simulink model "HILClimbers_LED_Rear_Light_Module_V5"  (R2021a)
settings: Solver=VariableStepAuto  StartTime=0.0  StopTime=inf  RelTol=1e-3
model workspace (MAT data in the model file):
  brake = 0
settings Model: Creator=Sai229  LastModifiedBy=Sai229

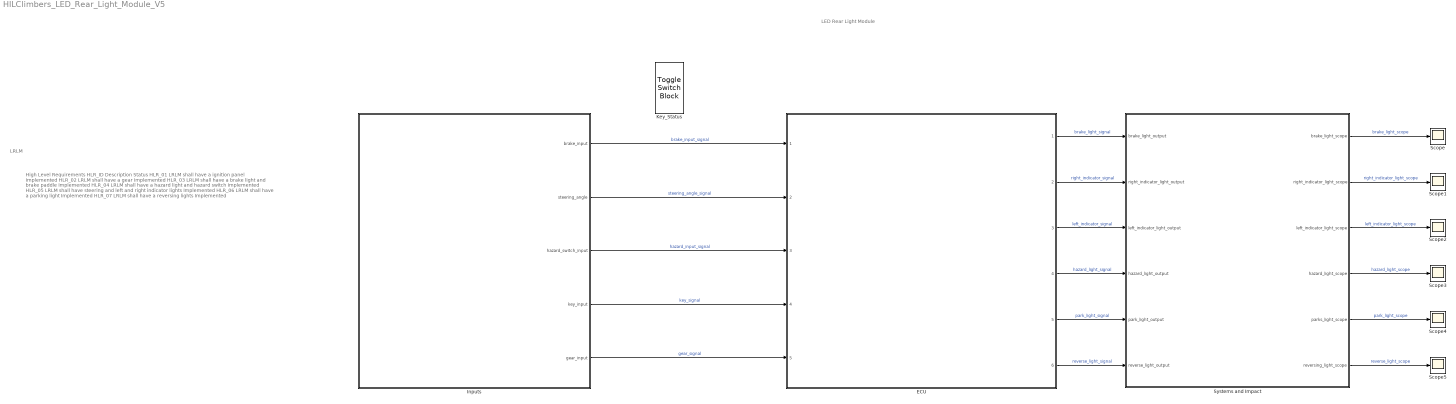
== system HILClimbers_LED_Rear_Light_Module_V5 ==
  note: LRLM
  note: High Level Requirements
      |
      | HLR_ID
      | Description
      | Status
      |
      | HLR_01
      | LRLM shall have a ignition panel
      | Implemented
      |
      | HLR_02
      | LRLM shall have a gear
      | Implemented
      |
      | HLR_03
      | LRLM shall have a brake light and brake paddle
      | Implemented
      |
      | HLR_04
      | LRLM shall have a hazard light and hazard switch
      | Implemented
      |
      | HLR_05
      | LRLM shall have steering and left and right indicator lights
      | Implemented
      |
      | HLR_06
      | LRLM shall have a parking light
      | Implemented
      |
      | HLR_07
      | LRLM shall have a reversing lights
      | Implemented
  note: LED Rear Light Module
  ECU : Subsystem  ReferencedSubsystem=LRLM_ECU
  Inputs : Subsystem
  Key_Status : ToggleSwitchBlock  LabelPosition=Hide
      settings: Values={{'Off', 'On'}, [0 1]}
  Scope{,1..5} (6 alike) : Scope
  Systems and Impact : Subsystem
  wires:
  Inputs/1(brake_input) -> ECU/1  "brake_input_signal"
  Inputs/2(steering_angle) -> ECU/2  "steering_angle_signal"
  Inputs/3(hazard_switch_input) -> ECU/3  "hazard_input_signal"
  Inputs/4(key_input) -> ECU/4  "key_signal"
  Inputs/5(gear_input) -> ECU/5  "gear_signal"
  ECU/1 -> Systems and Impact/1(brake_light_output)  "brake_light_signal"
  ECU/2 -> Systems and Impact/2(right_indicator_light_output)  "right_indicator_signal"
  ECU/3 -> Systems and Impact/3(left_indicator_light_output)  "left_indicator_signal"
  ECU/4 -> Systems and Impact/4(hazard_light_output)  "hazard_light_signal"
  ECU/5 -> Systems and Impact/5(park_light_output)  "park_light_signal"
  ECU/6 -> Systems and Impact/6(reverse_light_output)  "reverse_light_signal"
  Systems and Impact/1(brake_light_scope) -> Scope/1  "brake_light_scope"
  Systems and Impact/3(left_indicator_light_scope) -> Scope2/1  "left_indicator_light_scope"
  Systems and Impact/4(hazard_light_scope) -> Scope3/1  "hazard_light_scope"
  Systems and Impact/5(parks_light_scope) -> Scope4/1  "park_light_scope"
  Systems and Impact/6(reversing_light_scope) -> Scope5/1  "reverse_light_scope"
  Systems and Impact/2(right_indicator_light_scope) -> Scope1/1  "right_indicator_light_scope"

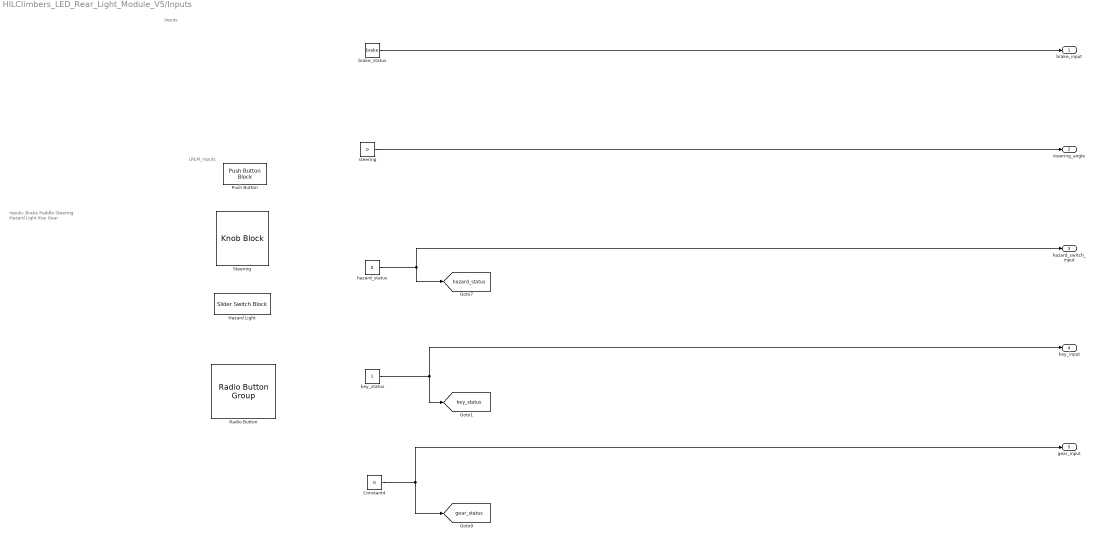
== system HILClimbers_LED_Rear_Light_Module_V5/Inputs ==
  note: Inputs
  note: LRLM_inputs
  note: Inputs:
      | Brake Paddle
      | Steering
      | Hazard Light
      | Key
      | Gear
  Constant4 : Constant  Value=0
  Hazard Light : SliderSwitchBlock  LabelPosition=Hide
      settings: Values={{'Off', 'On'}, [0 1]}
  Push Button : PushButtonBlock  ButtonText=Brake
  Radio Button : RadioButtonGroup  LabelPosition=Hide  SelectedLabel=Neutral  ButtonGroupName=Gear
      settings: Values={{'Neutral', 'Drive', 'Park', 'Reverse'}, [0 1 2 3]}
  Steering : KnobBlock  LabelPosition=Hide  ScaleMin=-50  ScaleMax=50  TickInterval=10
  brake_status : Constant  Value=brake
  hazard_status : Constant  Value=0
  key_status : Constant
  steering : Constant  Value=0
  brake_input : Outport
  steering_angle : Outport  Port=2
  hazard_switch_input : Outport  Port=3
  key_input : Outport  Port=4
  gear_input : Outport  Port=5
  tag scope: gear_status=global, hazard_status=global, key_status=global
  wires:
  brake_status/1 -> brake_input/1
  Constant4/1 -> [gear_status], gear_input/1
  steering/1 -> steering_angle/1
  key_status/1 -> [key_status], key_input/1
  hazard_status/1 -> hazard_switch_input/1, [hazard_status]

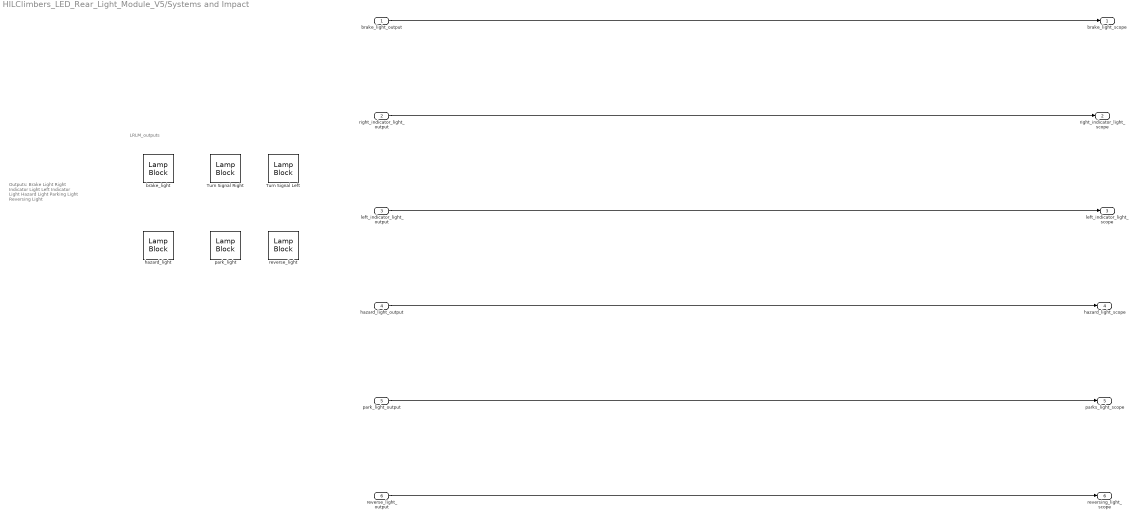
== system HILClimbers_LED_Rear_Light_Module_V5/Systems and Impact ==
  note: Outputs:
      | Brake Light
      | Right Indicator Light
      | Left Indicator Light
      | Hazard Light
      | Parking Light
      | Reversing Light
  note: LRLM_outputs
  brake_light_output : Inport
  right_indicator_light_output : Inport  Port=2
  left_indicator_light_output : Inport  Port=3
  hazard_light_output : Inport  Port=4
  park_light_output : Inport  Port=5
  reverse_light_output : Inport  Port=6
  Turn Signal Left : LampBlock  LabelPosition=Hide  Icon=TurnSignalLeft
  Turn Signal Right : LampBlock  LabelPosition=Hide  Icon=TurnSignalRight
  brake_light : LampBlock  LabelPosition=Hide  Icon=LightingSwitch
  hazard_light : LampBlock  LabelPosition=Hide  Icon=Hazards
  park_light : LampBlock  Icon=ParkingAssistance
  reverse_light : LampBlock  Icon=RearFogLight
  brake_light_scope : Outport
  right_indicator_light_scope : Outport  Port=2
  left_indicator_light_scope : Outport  Port=3
  hazard_light_scope : Outport  Port=4
  parks_light_scope : Outport  Port=5
  reversing_light_scope : Outport  Port=6
  wires:
  hazard_light_output/1 -> hazard_light_scope/1
  reverse_light_output/1 -> reversing_light_scope/1
  park_light_output/1 -> parks_light_scope/1
  left_indicator_light_output/1 -> left_indicator_light_scope/1
  right_indicator_light_output/1 -> right_indicator_light_scope/1
  brake_light_output/1 -> brake_light_scope/1
